simulink model "Simulacionoporedjenje"  (R2015a)
settings: Solver=ode3  StartTime=0.0  StopTime=50  FixedStep=0.01  RelTol=1e-3
settings Model: CovModelRefEnable=off  Creator=Avdo1  LastModifiedBy=PC
settings DataIOCC: SaveFormat=StructureWithTime
settings HardwareCC: ProdBitPerPointer=64  ProdLargestAtomicFloat=Float  ProdIntDivRoundTo=Zero  ProdEndianess=LittleEndian  ProdHWDeviceType=Specified
settings GRTTargetCC: GeneratePreprocessorConditionals=Use local settings

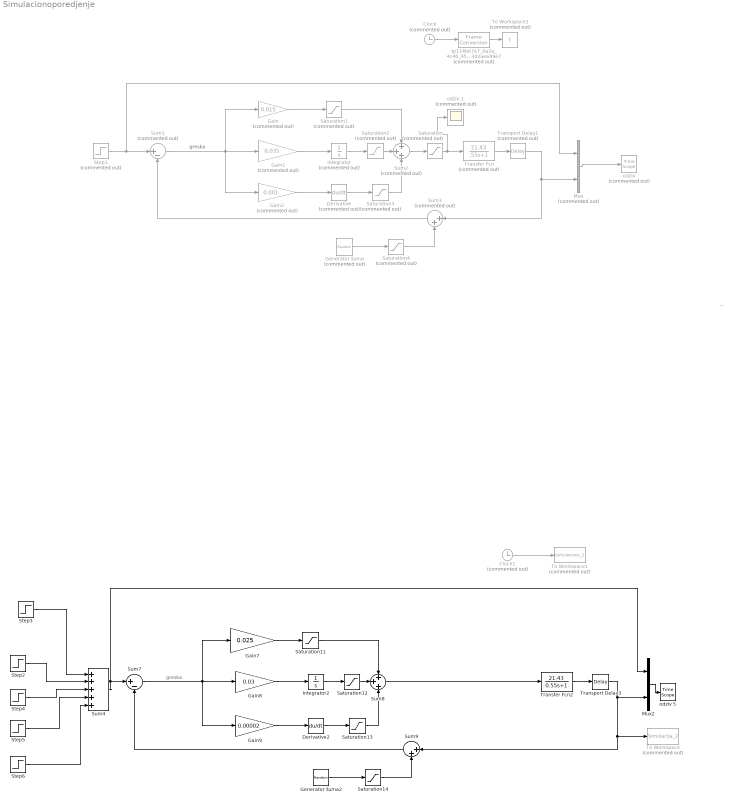
== system Simulacionoporedjenje ==
  note: --
  note: greska
  note: greska
  Clock : Clock  Commented=on
  Clock1 : Clock  Commented=on
  Derivative : Derivative  Commented=on
  Derivative2 : Derivative
  Gain : Gain  Commented=on  Gain=0.015
  Gain1 : Gain  Commented=on  Gain=0.035
  Gain2 : Gain  Commented=on  Gain=0.001
  Gain7 : Gain  Gain=0.025
  Gain8 : Gain  Gain=0.03
  Gain9 : Gain  Gain=0.00002
  Generator šuma : UniformRandomNumber  Commented=on  Minimum=0  Maximum=0.18  Seed=1  SampleTime=0.01
  Generator šuma2 : UniformRandomNumber  Minimum=0  Maximum=0.5  Seed=1  SampleTime=0.01
  Integrator : Integrator  Commented=on  LimitOutput=on  UpperSaturationLimit=10  LowerSaturationLimit=0
  Integrator2 : Integrator  LimitOutput=on  UpperSaturationLimit=10  LowerSaturationLimit=0
  Mux : Mux  Commented=on  Inputs=2
  Mux2 : Mux  Inputs=2
  Saturation{,1..4} (5 alike) : Saturate  Commented=on  UpperLimit=10  LowerLimit=0
  Saturation{11..14} (4 alike) : Saturate  UpperLimit=10  LowerLimit=0
  Step1 : Step  Commented=on  After=214  SampleTime=0
  Step2 : Step  Time=21.44  After=68.05  SampleTime=0
  Step3 : Step  Time=4.737  After=53.25  SampleTime=0
  Step4 : Step  Time=27.14  After=53.3  SampleTime=0
  Step5 : Step  Time=32.19  After=39.4  SampleTime=0
  Step6 : Step  Time=37.06  After=-104.5  SampleTime=0
  Sum1 : Sum  Commented=on  Inputs=|+-
  Sum2 : Sum  Commented=on  Inputs=+++
  Sum3 : Sum  Commented=on  Inputs=|++
  Sum4 : Sum  Inputs=+++++
  Sum7 : Sum  Inputs=|+-
  Sum8 : Sum  Inputs=+++
  Sum9 : Sum  Inputs=|++
  To Workspace : ToWorkspace  Commented=on  VariableName=Simulacija_2  SampleTime=-1
      settings: Save2DSignal=2-D array (concatenate along first dimension)
  To Workspace1 : ToWorkspace  Commented=on  VariableName=tsimulaciono_2  SampleTime=-1
      settings: Save2DSignal=2-D array (concatenate along first dimension)
  To Workspace2 : ToWorkspace  Commented=on  VariableName=t  SampleTime=-1
  Transfer Fcn : TransferFcn  Commented=on  Numerator=[21.43]  Denominator=[.55 1]
  Transfer Fcn2 : TransferFcn  Numerator=[21.43]  Denominator=[0.55 1]
  Transport Delay1 : TransportDelay  Commented=on  DelayTime=0.1
  Transport Delay3 : TransportDelay  DelayTime=0.1
  "odziv " : TimeScope  Commented=on
  odziv 1 : Scope  Commented=on
      settings: YMin=-1.25  YMax=11.25
  odziv 5 : TimeScope
  tp114b67e7_0a2a_4c40_9534_833d2ae699e7 : FrameConversion  Commented=on  OutFrame=Sample-based
  wires:
  Transfer Fcn/1 -> Transport Delay1/1
  Step1/1 -> Mux/1, Sum1/1
  Transport Delay1/1 -> Mux/2, Sum3/1
  Sum1/1 -> Gain2/1, Gain1/1, Gain/1
  Gain/1 -> Saturation1/1
  Sum2/1 -> Saturation/1
  Saturation/1 -> odziv 1/1, Transfer Fcn/1
  Sum3/1 -> Sum1/2
  Generator šuma/1 -> Saturation4/1
  Gain1/1 -> Integrator/1
  Gain2/1 -> Derivative/1
  Integrator/1 -> Saturation2/1
  Derivative/1 -> Saturation3/1
  Mux/1 -> "odziv "/1
  Saturation1/1 -> Sum2/1
  Saturation2/1 -> Sum2/2
  Saturation3/1 -> Sum2/3
  Saturation4/1 -> Sum3/2
  Clock/1 -> tp114b67e7_0a2a_4c40_9534_833d2ae699e7/1
  tp114b67e7_0a2a_4c40_9534_833d2ae699e7/1 -> To Workspace2/1
  Transfer Fcn2/1 -> Transport Delay3/1
  Transport Delay3/1 -> To Workspace/1, Sum9/1, Mux2/2
  Sum7/1 -> Gain9/1, Gain8/1, Gain7/1
  Gain7/1 -> Saturation11/1
  Sum9/1 -> Sum7/2
  Generator šuma2/1 -> Saturation14/1
  Gain8/1 -> Integrator2/1
  Gain9/1 -> Derivative2/1
  Integrator2/1 -> Saturation12/1
  Derivative2/1 -> Saturation13/1
  Mux2/1 -> odziv 5/1
  Saturation11/1 -> Sum8/1
  Saturation12/1 -> Sum8/2
  Saturation13/1 -> Sum8/3
  Saturation14/1 -> Sum9/2
  Sum8/1 -> Transfer Fcn2/1
  Sum4/1 -> Mux2/1, Sum7/1
  Step3/1 -> Sum4/1
  Step2/1 -> Sum4/2
  Step4/1 -> Sum4/3
  Step5/1 -> Sum4/4
  Clock1/1 -> To Workspace1/1
  Step6/1 -> Sum4/5
